simulink model "lab2p2"  (R2023b)
settings: Solver=ode3  StartTime=0.0  StopTime=Tmdl  FixedStep=To/100  RelTol=1e-3
undefined symbols (not defined in the file): an, dsc, To
settings Model: Creator=deniskirbaba  LastModifiedBy=deniskirbaba

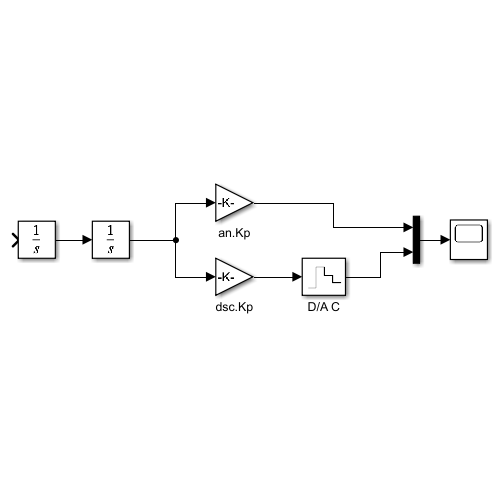
[thumbnail: Simulink's stored preview of the top-level diagram]
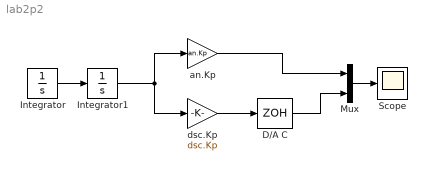
== system lab2p2 ==
  D/A C : ZeroOrderHold  SampleTime=To
  Integrator : Integrator  InitialCondition=1
  Integrator1 : Integrator
  Mux : Mux  Inputs=2
  Scope : Scope
  an.Kp : Gain  Gain=an.Kp
  dsc.Kp : Gain  Gain=dsc.Kp
  wires:
  dsc.Kp/1 -> D/A C/1
  Integrator1/1 -> dsc.Kp/1, an.Kp/1
  an.Kp/1 -> Mux/1
  D/A C/1 -> Mux/2
  Mux/1 -> Scope/1
  Integrator/1 -> Integrator1/1
